simulink library "Pitch_Actuation_Linkage_Lib"  (R2026a)
settings: Solver=ode45  EnableMultiTasking=on
Description:
  | Copyright 2009-2026 The MathWorks, Inc. MathWorks, Inc.
settings Model: Creator=smiller  LastModifiedBy=smiller
settings DataIOCC: SignalLoggingSaveFormat=ModelDataLogs
settings DebuggingCC: UnderspecifiedInitializationDetection=Classic  PregeneratedLibrarySubsystemCodeDiagnostic=none
settings HardwareCC: ProdHWDeviceType=32-bit Generic
settings GRTTargetCC: CombineOutputUpdateFcns=off  GRTInterface=on

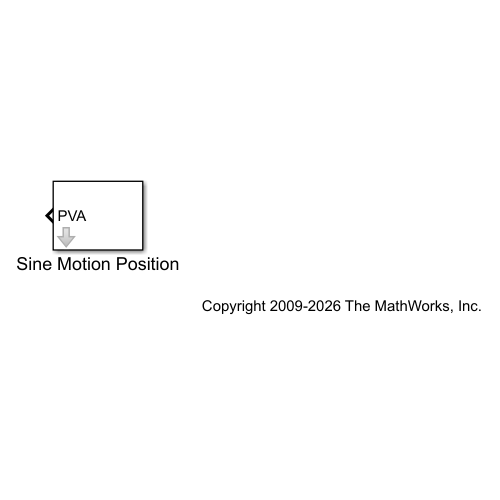
[thumbnail: Simulink's stored preview of the top-level diagram]
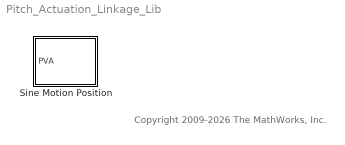
== system Pitch_Actuation_Linkage_Lib ==
  note: Copyright 2009-2026 The MathWorks, Inc.
  Sine Motion Position : Subsystem  mask{Amplitude=0.2, pd=5, PhaseShift=0}
      mask prompts: pd "Period (Seconds)"; PhaseShift "Phase Shift (Degrees)"

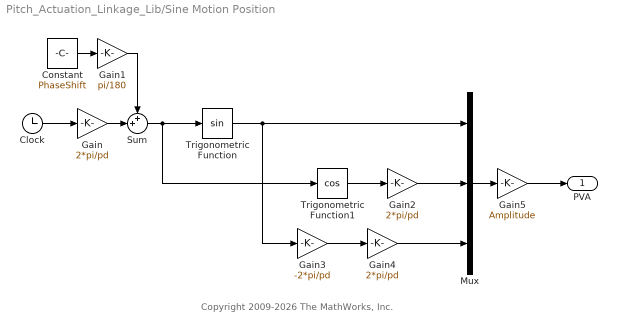
== system Pitch_Actuation_Linkage_Lib/Sine Motion Position ==
  note: Copyright 2009-2026 The MathWorks, Inc.
  Clock : Clock
  Constant : Constant  Value=PhaseShift
  Gain : Gain  Gain=2*pi/pd
  Gain1 : Gain  Gain=pi/180
  Gain2 : Gain  Gain=2*pi/pd
  Gain3 : Gain  Gain=-2*pi/pd
  Gain4 : Gain  Gain=2*pi/pd
  Gain5 : Gain  Gain=Amplitude
  Mux : Mux  Inputs=3
  Sum : Sum  Inputs=++|
  Trigonometric Function : Trigonometry
  Trigonometric Function1 : Trigonometry  Operator=cos
  PVA : Outport  VectorParamsAs1DForOutWhenUnconnected=off
  wires:
  Gain4/1 -> Mux/3
  Gain3/1 -> Gain4/1
  Gain2/1 -> Mux/2
  Trigonometric Function1/1 -> Gain2/1
  Gain5/1 -> PVA/1
  Mux/1 -> Gain5/1
  Trigonometric Function/1 -> Gain3/1, Mux/1
  Sum/1 -> Trigonometric Function1/1, Trigonometric Function/1
  Gain1/1 -> Sum/1
  Constant/1 -> Gain1/1
  Gain/1 -> Sum/2
  Clock/1 -> Gain/1
